simulink model "Simulink_DB"  (R2013a)
settings: Solver=ode3  StartTime=0.0  StopTime=inf  FixedStep=0.001  RelTol=1e-3
undefined symbols (not defined in the file or in its folder): d, NULL, serial
libraries: simulink x7, xpcseriallib x7, instrumentlib x2
settings Model: Creator=Petito  LastModifiedBy=Petito
settings HardwareCC: ProdIntDivRoundTo=Zero  ProdEndianess=LittleEndian  ProdHWDeviceType=Generic->32-bit x86 compatible
settings RTWCC: SystemTargetFile=rtwin.tlc  TemplateMakefile=rtwin.tmf  Description=Real-Time Windows Target  ProcessScript=rtwin_make_rtw_hook  RTWCompilerOptimization=On
settings CodeAppCC: MaxIdLength=95
settings RTWinTargetCC: TargetLibSuffix=_rtwin.lib  TargetPreCompLibLocation=C:\Program Files\MATLAB\R2013a\toolbox\rtw\targets\rtwin\lib\win64  CodeReplacementLibrary=ANSI_C  RTWinDir=C:/PROGRA~1/MATLAB/R2013a/toolbox/rtw/targets/rtwin  TargetArch=win64

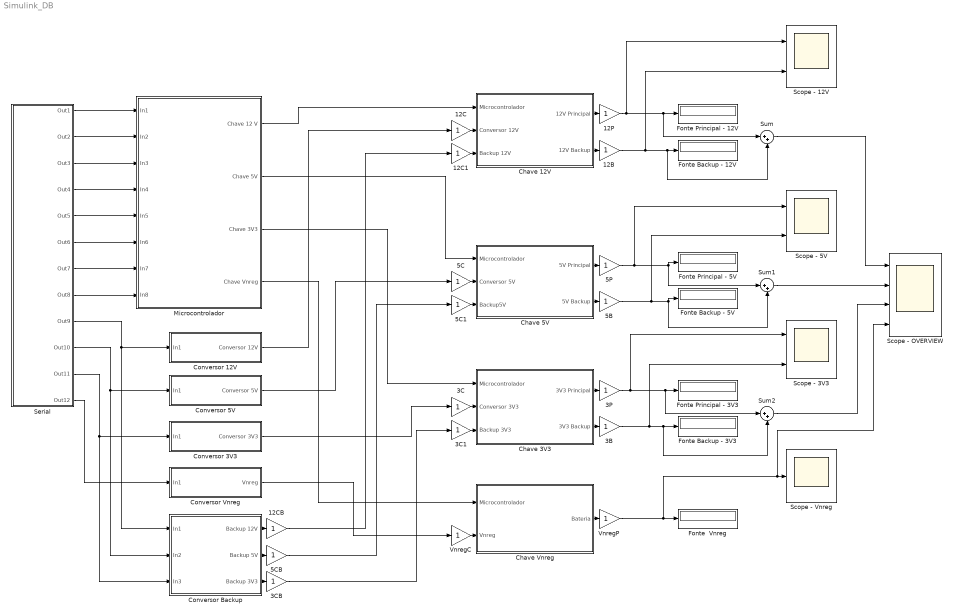
== system Simulink_DB ==
  12B : Gain
  12C : Gain
  12C1 : Gain
  12CB : Gain
  12P : Gain
  3B : Gain
  3C : Gain
  3C1 : Gain
  3CB : Gain
  3P : Gain
  5B : Gain
  5C : Gain
  5C1 : Gain
  5CB : Gain
  5P : Gain
  Chave 12V : Subsystem
  Chave 3V3 : Subsystem
  Chave 5V : Subsystem
  Chave Vnreg : Subsystem
  Conversor 12V : Subsystem
  Conversor 3V3 : Subsystem
  Conversor 5V : Subsystem
  Conversor Backup : Subsystem
  Conversor Vnreg : Subsystem
  Fonte  Vnreg : Display  mask(a){}
  Fonte Backup - 12V : Display
  Fonte Backup - 3V3 : Display
  Fonte Backup - 5V : Display
  Fonte Principal - 12V : Display  mask(a){}
  Fonte Principal - 3V3 : Display  mask(a){}
  Fonte Principal - 5V : Display  mask(a){}
  Microcontrolador : Subsystem
  Scope - 12V : Scope  NumInputPorts=2
      settings: TickLabels=on  TimeRange=10  YMin=0~0  YMax=13~13
  Scope - 3V3 : Scope  NumInputPorts=2
      settings: TickLabels=on  TimeRange=10  YMin=0~0  YMax=13~13  SaveName=ScopeData3
  Scope - 5V : Scope  NumInputPorts=2
      settings: TickLabels=on  TimeRange=10  YMin=0~0  YMax=6~6.5  SaveName=ScopeData2
  Scope - OVERVIEW : Scope  NumInputPorts=4
      settings: TickLabels=on  TimeRange=10  YMin=0~0~0~0  YMax=13~6~4~9
  Scope - Vnreg : Scope
      settings: TickLabels=on  TimeRange=10  YMin=0  YMax=13  SaveName=ScopeData4
  Serial : Subsystem
  Sum : Sum  Inputs=|++
  Sum1 : Sum  Inputs=|++
  Sum2 : Sum  Inputs=|++
  VnregC : Gain
  VnregP : Gain
  wires:
  Microcontrolador/3(Chave 3V3) -> Chave 3V3/1(Microcontrolador)
  Conversor 3V3/1(Conversor 3V3) -> 3C/1
  Conversor Backup/3(Backup 3V3) -> 3CB/1
  Microcontrolador/2(Chave 5V) -> Chave 5V/1(Microcontrolador)
  Conversor 5V/1(Conversor 5V) -> 5C/1
  Conversor Backup/2(Backup 5V) -> 5CB/1
  Conversor 12V/1(Conversor 12V) -> 12C/1
  Conversor Backup/1(Backup 12V) -> 12CB/1
  Conversor Vnreg/1(Vnreg) -> VnregC/1
  Microcontrolador/4(Chave Vnreg) -> Chave Vnreg/1(Microcontrolador)
  Chave Vnreg/1(Bateria) -> VnregP/1
  Chave 3V3/1(3V3 Principal) -> 3P/1
  Chave 3V3/2(3V3 Backup) -> 3B/1
  Chave 5V/1(5V Principal) -> 5P/1
  Chave 5V/2(5V Backup) -> 5B/1
  Chave 12V/2(12V Backup) -> 12B/1
  Microcontrolador/1(Chave 12 V) -> Chave 12V/1(Microcontrolador)
  Chave 12V/1(12V Principal) -> 12P/1
  12P/1 -> Scope - 12V/1, Fonte Principal - 12V/1, Sum/1
  12B/1 -> Scope - 12V/2, Sum/2, Fonte Backup - 12V/1
  5P/1 -> Scope - 5V/1, Fonte Principal - 5V/1, Sum1/1
  5B/1 -> Scope - 5V/2, Fonte Backup - 5V/1, Sum1/2
  VnregP/1 -> Scope - OVERVIEW/4, Scope - Vnreg/1, Fonte  Vnreg/1
  Serial/1(Out1) -> Microcontrolador/1(In1)
  Serial/2(Out2) -> Microcontrolador/2(In2)
  Serial/3(Out3) -> Microcontrolador/3(In3)
  Serial/4(Out4) -> Microcontrolador/4(In4)
  Serial/5(Out5) -> Microcontrolador/5(In5)
  Serial/6(Out6) -> Microcontrolador/6(In6)
  Serial/7(Out7) -> Microcontrolador/7(In7)
  Serial/8(Out8) -> Microcontrolador/8(In8)
  Serial/9(Out9) -> Conversor Backup/1(In1), Conversor 12V/1(In1)
  Serial/10(Out10) -> Conversor Backup/2(In2), Conversor 5V/1(In1)
  Serial/11(Out11) -> Conversor Backup/3(In3), Conversor 3V3/1(In1)
  Serial/12(Out12) -> Conversor Vnreg/1(In1)
  12C/1 -> Chave 12V/2(Conversor 12V)
  5C/1 -> Chave 5V/2(Conversor 5V)
  3C/1 -> Chave 3V3/2(Conversor 3V3)
  VnregC/1 -> Chave Vnreg/2(Vnreg)
  12CB/1 -> 12C1/1
  5CB/1 -> 5C1/1
  3CB/1 -> 3C1/1
  12C1/1 -> Chave 12V/3(Backup 12V)
  5C1/1 -> Chave 5V/3(Backup5V)
  3C1/1 -> Chave 3V3/3(Backup 3V3)
  Sum/1 -> Scope - OVERVIEW/1
  Sum1/1 -> Scope - OVERVIEW/2
  3P/1 -> Scope - 3V3/1, Sum2/1, Fonte Principal - 3V3/1
  3B/1 -> Scope - 3V3/2, Sum2/2, Fonte Backup - 3V3/1
  Sum2/1 -> Scope - OVERVIEW/3

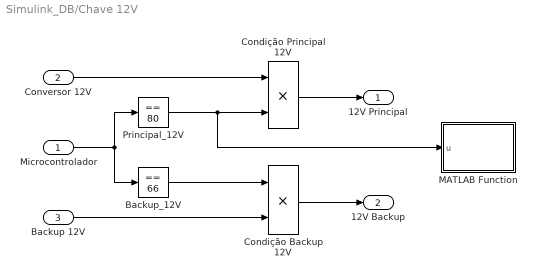
== system Simulink_DB/Chave 12V ==
  Microcontrolador : Inport
  Conversor 12V : Inport  Port=2
  Backup 12V : Inport  Port=3
  Backup_12V : simulink/Logic and Bit Operations/Compare To Constant  relop===  const=66  OutDataTypeStr=boolean
  Condição Backup 12V : Product
  Condição Principal 12V : Product
  MATLAB Function : MATLAB Function  TreatAsAtomicUnit=on
  Principal_12V : simulink/Logic and Bit Operations/Compare To Constant  relop===  const=80  OutDataTypeStr=boolean
  12V Principal : Outport
  12V Backup : Outport  Port=2
  wires:
  Microcontrolador/1 -> Principal_12V/1, Backup_12V/1
  Principal_12V/1 -> MATLAB Function/1(u), Condição Principal 12V/2
  Conversor 12V/1 -> Condição Principal 12V/1
  Backup_12V/1 -> Condição Backup 12V/1
  Backup 12V/1 -> Condição Backup 12V/2
  Condição Principal 12V/1 -> 12V Principal/1
  Condição Backup 12V/1 -> 12V Backup/1

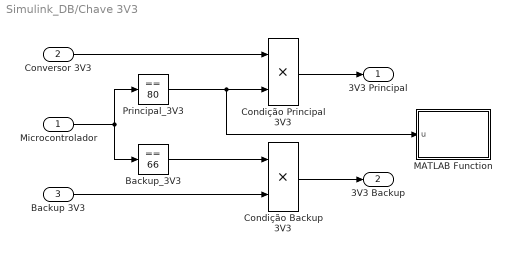
== system Simulink_DB/Chave 3V3 ==
  Microcontrolador : Inport
  Conversor 3V3 : Inport  Port=2
  Backup 3V3 : Inport  Port=3
  Backup_3V3 : simulink/Logic and Bit Operations/Compare To Constant  relop===  const=66  OutDataTypeStr=boolean
  Condição Backup 3V3 : Product
  Condição Principal 3V3 : Product
  MATLAB Function : MATLAB Function  TreatAsAtomicUnit=on
  Principal_3V3 : simulink/Logic and Bit Operations/Compare To Constant  relop===  const=80  OutDataTypeStr=boolean
  3V3 Principal : Outport
  3V3 Backup : Outport  Port=2
  wires:
  Microcontrolador/1 -> Principal_3V3/1, Backup_3V3/1
  Principal_3V3/1 -> MATLAB Function/1(u), Condição Principal 3V3/2
  Conversor 3V3/1 -> Condição Principal 3V3/1
  Backup_3V3/1 -> Condição Backup 3V3/1
  Backup 3V3/1 -> Condição Backup 3V3/2
  Condição Principal 3V3/1 -> 3V3 Principal/1
  Condição Backup 3V3/1 -> 3V3 Backup/1

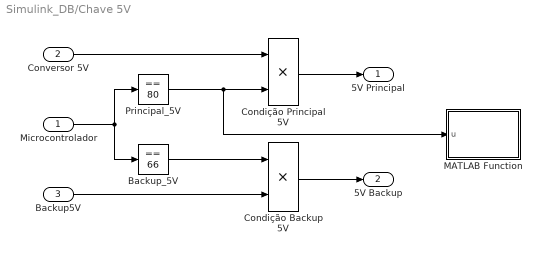
== system Simulink_DB/Chave 5V ==
  Microcontrolador : Inport
  Conversor 5V : Inport  Port=2
  Backup5V : Inport  Port=3
  Backup_5V : simulink/Logic and Bit Operations/Compare To Constant  relop===  const=66  OutDataTypeStr=boolean
  Condição Backup 5V : Product
  Condição Principal 5V : Product
  MATLAB Function : MATLAB Function  TreatAsAtomicUnit=on
  Principal_5V : simulink/Logic and Bit Operations/Compare To Constant  relop===  const=80  OutDataTypeStr=boolean
  5V Principal : Outport
  5V Backup : Outport  Port=2
  wires:
  Microcontrolador/1 -> Principal_5V/1, Backup_5V/1
  Principal_5V/1 -> MATLAB Function/1(u), Condição Principal 5V/2
  Conversor 5V/1 -> Condição Principal 5V/1
  Backup_5V/1 -> Condição Backup 5V/1
  Backup5V/1 -> Condição Backup 5V/2
  Condição Principal 5V/1 -> 5V Principal/1
  Condição Backup 5V/1 -> 5V Backup/1

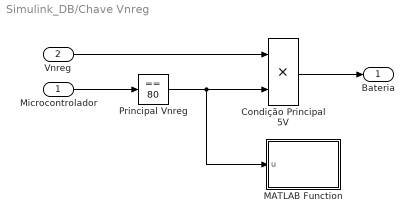
== system Simulink_DB/Chave Vnreg ==
  Microcontrolador : Inport
  Vnreg : Inport  Port=2
  Condição Principal 5V : Product
  MATLAB Function : MATLAB Function  TreatAsAtomicUnit=on
  Principal Vnreg : simulink/Logic and Bit Operations/Compare To Constant  relop===  const=80  OutDataTypeStr=boolean
  Bateria : Outport
  wires:
  Microcontrolador/1 -> Principal Vnreg/1
  Principal Vnreg/1 -> MATLAB Function/1(u), Condição Principal 5V/2
  Vnreg/1 -> Condição Principal 5V/1
  Condição Principal 5V/1 -> Bateria/1

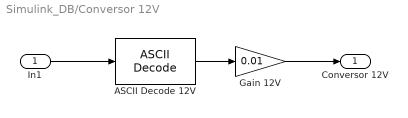
== system Simulink_DB/Conversor 12V ==
  In1 : Inport
  "ASCII Decode 12V " : xpcseriallib/ASCII Decode   format=%d\0  nvars=1  vartypes={}
  Gain 12V : Gain  Gain=0.01  ParamMin=[0]
  Conversor 12V : Outport
  wires:
  "ASCII Decode 12V "/1 -> Gain 12V/1
  In1/1 -> "ASCII Decode 12V "/1
  Gain 12V/1 -> Conversor 12V/1

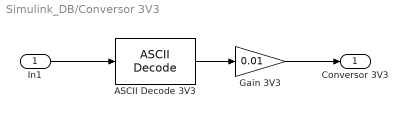
== system Simulink_DB/Conversor 3V3 ==
  In1 : Inport
  "ASCII Decode 3V3 " : xpcseriallib/ASCII Decode   format=%d\0  nvars=1  vartypes={}
  Gain 3V3 : Gain  Gain=0.01  ParamMin=[0]
  Conversor 3V3 : Outport
  wires:
  "ASCII Decode 3V3 "/1 -> Gain 3V3/1
  In1/1 -> "ASCII Decode 3V3 "/1
  Gain 3V3/1 -> Conversor 3V3/1

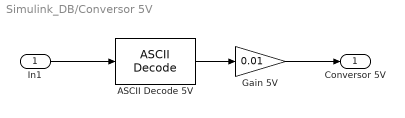
== system Simulink_DB/Conversor 5V ==
  In1 : Inport
  "ASCII Decode 5V " : xpcseriallib/ASCII Decode   format=%d\0  nvars=1  vartypes={}
  Gain 5V : Gain  Gain=0.01  ParamMin=[0]
  Conversor 5V : Outport
  wires:
  "ASCII Decode 5V "/1 -> Gain 5V/1
  In1/1 -> "ASCII Decode 5V "/1
  Gain 5V/1 -> Conversor 5V/1

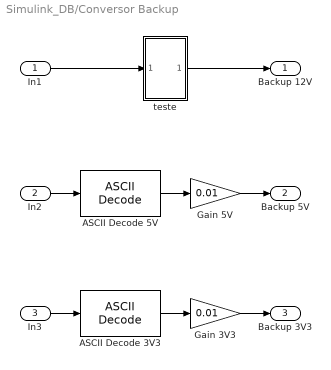
== system Simulink_DB/Conversor Backup ==
  In1 : Inport
  In2 : Inport  Port=2
  In3 : Inport  Port=3
  ASCII Decode 3V3 : xpcseriallib/ASCII Decode   format=%d\0  nvars=1  vartypes={}
  ASCII Decode 5V : xpcseriallib/ASCII Decode   format=%d\0  nvars=1  vartypes={}
  Gain 3V3 : Gain  Gain=0.01  ParamMin=[0]
  Gain 5V : Gain  Gain=0.01  ParamMin=[0]
  teste : Subsystem
  Backup 12V : Outport
  Backup 5V : Outport  Port=2
  Backup 3V3 : Outport  Port=3
  wires:
  ASCII Decode 5V/1 -> Gain 5V/1
  In2/1 -> ASCII Decode 5V/1
  Gain 5V/1 -> Backup 5V/1
  ASCII Decode 3V3/1 -> Gain 3V3/1
  In3/1 -> ASCII Decode 3V3/1
  Gain 3V3/1 -> Backup 3V3/1
  In1/1 -> teste/1(In1)
  teste/1(Out1) -> Backup 12V/1

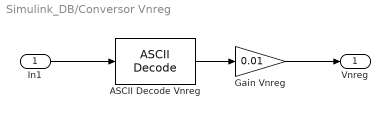
== system Simulink_DB/Conversor Vnreg ==
  In1 : Inport
  "ASCII Decode Vnreg " : xpcseriallib/ASCII Decode   format=%d\0  nvars=1  vartypes={}
  Gain Vnreg : Gain  Gain=0.01  ParamMin=[0]
  Vnreg : Outport
  wires:
  "ASCII Decode Vnreg "/1 -> Gain Vnreg/1
  In1/1 -> "ASCII Decode Vnreg "/1
  Gain Vnreg/1 -> Vnreg/1

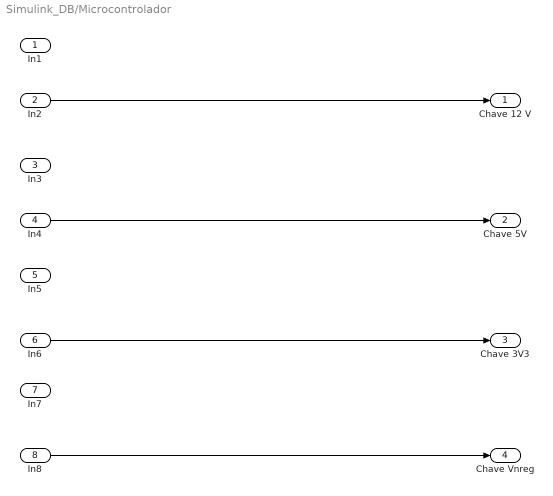
== system Simulink_DB/Microcontrolador ==
  In1 : Inport
  In2 : Inport  Port=2
  In3 : Inport  Port=3
  In4 : Inport  Port=4
  In5 : Inport  Port=5
  In6 : Inport  Port=6
  In7 : Inport  Port=7
  In8 : Inport  Port=8
  Chave 12 V : Outport
  Chave 5V : Outport  Port=2
  Chave 3V3 : Outport  Port=3
  Chave Vnreg : Outport  Port=4
  wires:
  In4/1 -> Chave 5V/1
  In6/1 -> Chave 3V3/1
  In8/1 -> Chave Vnreg/1
  In2/1 -> Chave 12 V/1

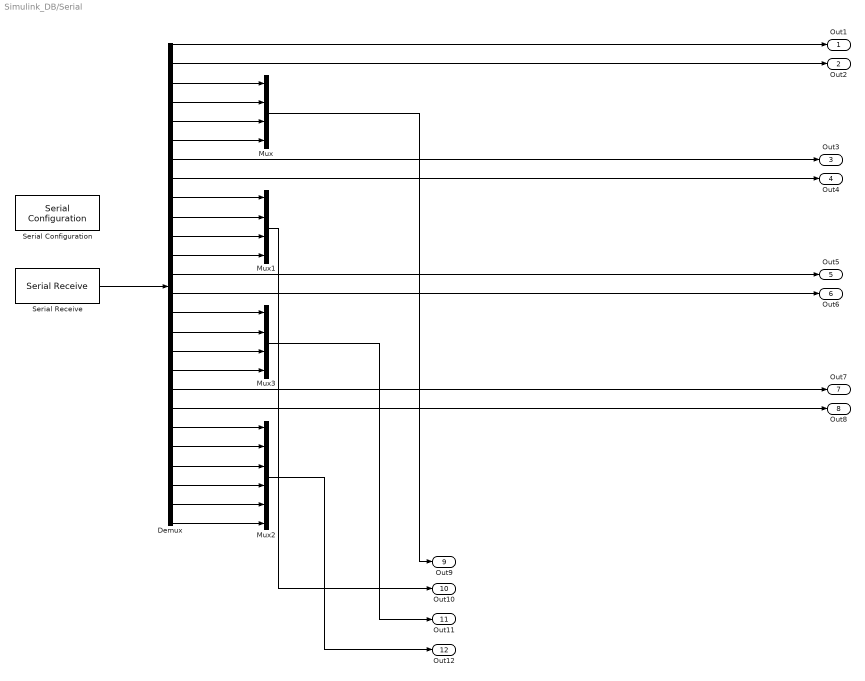
== system Simulink_DB/Serial ==
  Demux : Demux  Outputs=26
  Mux : Mux
  Mux1 : Mux
  Mux2 : Mux  Inputs=6
  Mux3 : Mux
  Serial Configuration : instrumentlib/Serial Configuration  Priority=-200000  ComPortMenu=<Please select a port...>  ComPort=COM7  ObjConstructor=serial('COM7');  BaudRate=9600  DataBits=8  Parity=none  StopBits=1  FlowControl=none  Timeout=10  ByteOrder=LittleEndian
  Serial Receive : instrumentlib/Serial Receive  ComPortMenu=<Please select a port...>  ComPort=COM7  ObjConstructor=serial('COM7');  Terminator=NULL ('\0')  DataSize="[1  26]"  DataType=int8  EnableBlockingMode=on  ActionDataUnavailable=Output last received value  CustomValue=0  SampleTime=0.01
  Out1 : Outport
  Out2 : Outport  Port=2
  Out3 : Outport  Port=3
  Out4 : Outport  Port=4
  Out5 : Outport  Port=5
  Out6 : Outport  Port=6
  Out7 : Outport  Port=7
  Out8 : Outport  Port=8
  Out9 : Outport  Port=9
  Out10 : Outport  Port=10
  Out11 : Outport  Port=11
  Out12 : Outport  Port=12
  wires:
  Mux3/1 -> Out11/1
  Demux/21 -> Mux2/1
  Demux/22 -> Mux2/2
  Demux/25 -> Mux2/5
  Demux/20 -> Out8/1
  Demux/13 -> Out5/1
  Mux1/1 -> Out10/1
  Mux/1 -> Out9/1
  Serial Receive/1 -> Demux/1
  Demux/26 -> Mux2/6
  Demux/24 -> Mux2/4
  Demux/23 -> Mux2/3
  Demux/10 -> Mux1/2
  Demux/17 -> Mux3/3
  Demux/18 -> Mux3/4
  Demux/12 -> Mux1/4
  Demux/5 -> Mux/3
  Demux/16 -> Mux3/2
  Demux/15 -> Mux3/1
  Demux/6 -> Mux/4
  Demux/9 -> Mux1/1
  Demux/4 -> Mux/2
  Demux/3 -> Mux/1
  Demux/11 -> Mux1/3
  Demux/2 -> Out2/1
  Demux/1 -> Out1/1
  Demux/8 -> Out4/1
  Demux/14 -> Out6/1
  Demux/19 -> Out7/1
  Demux/7 -> Out3/1
  Mux2/1 -> Out12/1

== system Simulink_DB/Conversor Backup/teste ==
  In1 : Inport
  "ASCII Decode 12V " : xpcseriallib/ASCII Decode   format=%d\0  nvars=1  vartypes={}
  Gain 12V : Gain  Gain=0.01  ParamMin=[0]
  Out1 : Outport
  wires:
  Gain 12V/1 -> Out1/1
  "ASCII Decode 12V "/1 -> Gain 12V/1
  In1/1 -> "ASCII Decode 12V "/1

== matlab function Simulink_DB/Chave 5V/MATLAB Function ==
  data: u input
function fcn(u)
%#codegen
coder.extrinsic('set_param');

set_param('Simulink_DB/Sum1','ForegroundColor','green');
set_param('Simulink_DB/Sum1','BackgroundColor','green');

if u > 0
    set_param('Simulink_DB/5P','BackgroundColor','green');
    set_param('Simulink_DB/5B','BackgroundColor','red');
    set_param('Simulink_DB/5P','ForegroundColor','green');
    set_param('Simulink_DB/5B','ForegroundColor','red');
    set_param('Simulink_DB/Conversor 5V','ForegroundColor','green');
    set_param('Simulink_DB/Conversor 5V','BackgroundColor','green');
    set_param('Simulink_DB/5C','BackgroundColor','green');
    set_param('Simulink_DB/5C','ForegroundColor','green');
    set_param('Simulink_DB/5C1','BackgroundColor','red');
    set_param('Simulink_DB/5CB','BackgroundColor','red');
    set_param('Simulink_DB/5C1','ForegroundColor','red');
    set_param('Simulink_DB/5CB','ForegroundColor','red');
else
    set_param('Simulink_DB/5P','BackgroundColor','red');
    set_param('Simulink_DB/5B','BackgroundColor','green');
    set_param('Simulink_DB/5P','ForegroundColor','red');
    set_param('Simulink_DB/5B','ForegroundColor','green');
    set_param('Simulink_DB/Conversor 5V','ForegroundColor','red');
    set_param('Simulink_DB/Conversor 5V','BackgroundColor','red');
    set_param('Simulink_DB/5C','BackgroundColor','red');
    set_param('Simulink_DB/5C','ForegroundColor','red');
    set_param('Simulink_DB/5C1','BackgroundColor','green');
    set_param('Simulink_DB/5CB','BackgroundColor','green');
    set_param('Simulink_DB/5C1','ForegroundColor','green');
    set_param('Simulink_DB/5CB','ForegroundColor','green');
end;

== matlab function Simulink_DB/Chave 12V/MATLAB Function ==
  data: u input
function fcn(u)
%#codegen
coder.extrinsic('set_param');

set_param('Simulink_DB/Sum','ForegroundColor','green');
set_param('Simulink_DB/Sum','BackgroundColor','green');

if u > 0
    set_param('Simulink_DB/12P','BackgroundColor','green');
    set_param('Simulink_DB/12P','ForegroundColor','green');
    set_param('Simulink_DB/12B','BackgroundColor','red');
    set_param('Simulink_DB/12B','ForegroundColor','red');
    set_param('Simulink_DB/Conversor 12V','ForegroundColor','green');
    set_param('Simulink_DB/Conversor 12V','BackgroundColor','green');
    set_param('Simulink_DB/12C','BackgroundColor','green');
    set_param('Simulink_DB/12C','ForegroundColor','green');
    set_param('Simulink_DB/12C1','BackgroundColor','red');
    set_param('Simulink_DB/12CB','BackgroundColor','red');
    set_param('Simulink_DB/12C1','ForegroundColor','red');
    set_param('Simulink_DB/12CB','ForegroundColor','red');
else
    set_param('Simulink_DB/12P','BackgroundColor','red');
    set_param('Simulink_DB/12B','BackgroundColor','green');
    set_param('Simulink_DB/12P','ForegroundColor','red');
    set_param('Simulink_DB/12B','ForegroundColor','green');
    set_param('Simulink_DB/Conversor 12V','ForegroundColor','red');
    set_param('Simulink_DB/Conversor 12V','BackgroundColor','red');
    set_param('Simulink_DB/12CB','BackgroundColor','green');
    set_param('Simulink_DB/12C','BackgroundColor','red');
    set_param('Simulink_DB/12C','ForegroundColor','red');
    set_param('Simulink_DB/12C1','BackgroundColor','green');
    set_param('Simulink_DB/12C1','ForegroundColor','green');
    set_param('Simulink_DB/12CB','ForegroundColor','green');
end;

== matlab function Simulink_DB/Chave 3V3/MATLAB Function ==
  data: u input
function fcn(u)
%#codegen
coder.extrinsic('set_param');

set_param('Simulink_DB/Sum2','ForegroundColor','green');
set_param('Simulink_DB/Sum2','BackgroundColor','green');


if u > 0
    set_param('Simulink_DB/3P','BackgroundColor','green');
    set_param('Simulink_DB/3P','ForegroundColor','green');
    set_param('Simulink_DB/3B','BackgroundColor','red');
    set_param('Simulink_DB/3B','ForegroundColor','red');
    set_param('Simulink_DB/Conversor 3V3','ForegroundColor','green');
    set_param('Simulink_DB/Conversor 3V3','BackgroundColor','green');
    set_param('Simulink_DB/3C','BackgroundColor','green');
    set_param('Simulink_DB/3C','ForegroundColor','green');
    set_param('Simulink_DB/3C1','BackgroundColor','red');
    set_param('Simulink_DB/3CB','BackgroundColor','red');
    set_param('Simulink_DB/3C1','ForegroundColor','red');
    set_param('Simulink_DB/3CB','ForegroundColor','red');
else
    set_param('Simulink_DB/3P','BackgroundColor','red');
    set_param('Simulink_DB/3P','ForegroundColor','red');
    set_param('Simulink_DB/3B','BackgroundColor','green');
    set_param('Simulink_DB/3B','ForegroundColor','green');
    set_param('Simulink_DB/Conversor 3V3','ForegroundColor','red');
    set_param('Simulink_DB/Conversor 3V3','BackgroundColor','red');
    set_param('Simulink_DB/3C','BackgroundColor','red');
    set_param('Simulink_DB/3C','ForegroundColor','red');
    set_param('Simulink_DB/3C1','BackgroundColor','green');
    set_param('Simulink_DB/3CB','BackgroundColor','green');
    set_param('Simulink_DB/3C1','ForegroundColor','green');
    set_param('Simulink_DB/3CB','ForegroundColor','green');
end;

== matlab function Simulink_DB/Chave Vnreg/MATLAB Function ==
  data: u input
function fcn(u)
%#codegen
coder.extrinsic('set_param');
if u > 0
    set_param('Simulink_DB/VnregP','BackgroundColor','green');
    set_param('Simulink_DB/VnregP','ForegroundColor','green');
    set_param('Simulink_DB/Conversor Vnreg','ForegroundColor','green');
    set_param('Simulink_DB/Conversor Vnreg','BackgroundColor','green');
    set_param('Simulink_DB/VnregC','BackgroundColor','green');
    set_param('Simulink_DB/VnregC','ForegroundColor','green');    
else
    set_param('Simulink_DB/VnregP','BackgroundColor','red');
    set_param('Simulink_DB/VnregP','ForegroundColor','red');
    set_param('Simulink_DB/Conversor Vnreg','ForegroundColor','red');
    set_param('Simulink_DB/Conversor Vnreg','BackgroundColor','red');
    set_param('Simulink_DB/VnregC','BackgroundColor','red');
    set_param('Simulink_DB/VnregC','ForegroundColor','red');
end;
